simulink model "filtered_deriv"  (Simulink 6.6)
settings: Solver=ode45  StartTime=0.0  StopTime=10.0  RelTol=1e-3
settings Model: Creator=yamokosk  LastModifiedBy=yamokosk  ExtModeAutoUpdateStatusClock=off

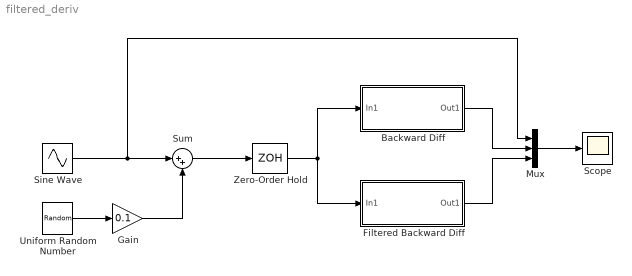
== system filtered_deriv ==
  Backward Diff : Subsystem
  Filtered Backward Diff : Subsystem
  Gain : Gain  Gain=0.1
  Mux : Mux  Inputs=3
  Scope : Scope
  Sine Wave : Sin  Amplitude=2  Frequency=2  SampleTime=0
  Sum : Sum  Inputs=|++
  Uniform Random Number : UniformRandomNumber  SampleTime=0
  Zero-Order Hold : ZeroOrderHold  SampleTime=0.01
  wires:
  Sine Wave/1 -> Sum/1, Mux/1
  Uniform Random Number/1 -> Gain/1
  Sum/1 -> Zero-Order Hold/1
  Zero-Order Hold/1 -> Backward Diff/1(In1), Filtered Backward Diff/1(In1)
  Mux/1 -> Scope/1
  Gain/1 -> Sum/2
  Filtered Backward Diff/1(Out1) -> Mux/3
  Backward Diff/1(Out1) -> Mux/2

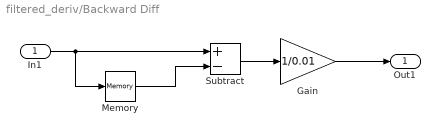
== system filtered_deriv/Backward Diff ==
  In1 : Inport
  Gain : Gain  Gain=1/0.01
  Memory : Memory  InheritSampleTime=on
  Subtract : Sum  Inputs=+-  OutScaling=2^-10
  Out1 : Outport
  wires:
  Subtract/1 -> Gain/1
  In1/1 -> Memory/1, Subtract/1
  Memory/1 -> Subtract/2
  Gain/1 -> Out1/1

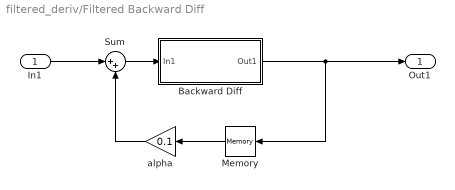
== system filtered_deriv/Filtered Backward Diff ==
  In1 : Inport
  Backward Diff : Subsystem
  Memory : Memory  Orientation=left  InheritSampleTime=on
  Sum : Sum  Inputs=|++
  alpha : Gain  Orientation=left  Gain=0.1
  Out1 : Outport
  wires:
  Memory/1 -> alpha/1
  In1/1 -> Sum/1
  alpha/1 -> Sum/2
  Sum/1 -> Backward Diff/1(In1)
  Backward Diff/1(Out1) -> Out1/1, Memory/1

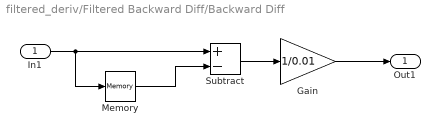
== system filtered_deriv/Filtered Backward Diff/Backward Diff ==
  In1 : Inport
  Gain : Gain  Gain=1/0.01
  Memory : Memory  InheritSampleTime=on
  Subtract : Sum  Inputs=+-  OutScaling=2^-10
  Out1 : Outport
  wires:
  Gain/1 -> Out1/1
  Memory/1 -> Subtract/2
  In1/1 -> Subtract/1, Memory/1
  Subtract/1 -> Gain/1
